simulink subsystem "Sensors"  (R2025a)
settings: Solver=VariableStepAuto  StartTime=0.0  StopTime=10.0  RelTol=1e-3
undefined symbols (not defined in the file): DiscIntNeverNeededParam, gyro_bias0, gyro_bias_rw, gyro_sigma, rng_seed, star_sigma, Ts_base, Ts_gyro, Ts_star
settings Model: Creator=Jackt  LastModifiedBy=Jackt

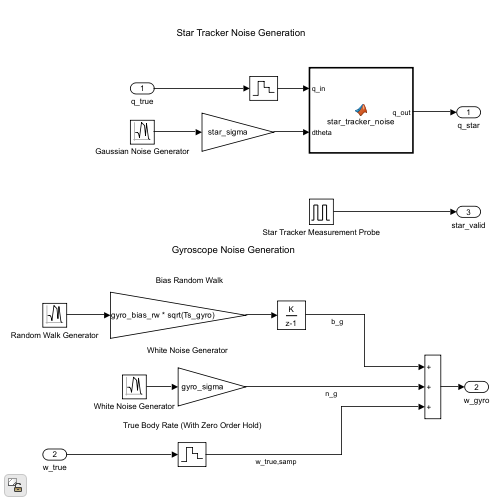
[thumbnail: Simulink's stored preview of the top-level diagram]
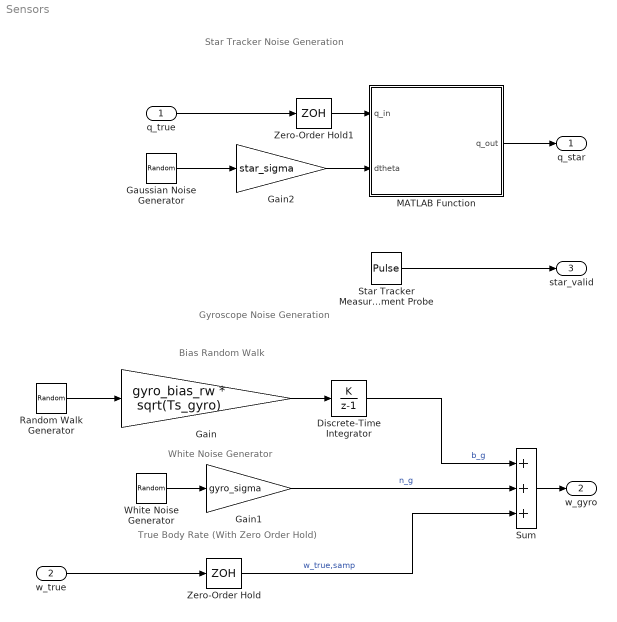
== system Sensors ==
  note: Gyroscope Noise Generation
  note: True Body Rate (With Zero Order Hold)
  note: White Noise Generator
  note: Bias Random Walk
  note: Star Tracker Noise Generation
  q_true : Inport
  w_true : Inport  Port=2
  Discrete-Time Integrator : DiscreteIntegrator  IntegratorMethod=Accumulation: Forward Euler  InitialCondition=gyro_bias0  SampleTime=Ts_gyro  ICPrevOutput=DiscIntNeverNeededParam  ICPrevScaledInput=DiscIntNeverNeededParam
  Gain : Gain  Gain=gyro_bias_rw * sqrt(Ts_gyro)
  Gain1 : Gain  Gain=gyro_sigma
  Gain2 : Gain  Gain=star_sigma
  Gaussian Noise Generator : RandomNumber  Mean=[0; 0; 0]  Variance=[1; 1; 1]  Seed=rng_seed  SampleTime=Ts_star  VectorParams1D=off
  MATLAB Function : MATLAB Function  TreatAsAtomicUnit=on
  Random Walk Generator : RandomNumber  Mean=[0; 0; 0]  Variance=[1; 1; 1]  Seed=rng_seed  SampleTime=Ts_gyro  VectorParams1D=off
  Star Tracker Measurement Probe : DiscretePulseGenerator  PulseType=Time based  Period=Ts_star  PulseWidth=100*Ts_base/Ts_star  VectorParams1D=off
  Sum : Sum  Inputs=+++
  White Noise Generator : RandomNumber  Mean=[0; 0; 0]  Variance=[1; 1; 1]  Seed=rng_seed  SampleTime=Ts_gyro  VectorParams1D=off
  Zero-Order Hold : ZeroOrderHold  SampleTime=Ts_gyro
  Zero-Order Hold1 : ZeroOrderHold  SampleTime=Ts_star
  q_star : Outport
  w_gyro : Outport  Port=2
  star_valid : Outport  Port=3
  wires:
  q_true/1 -> Zero-Order Hold1/1
  w_true/1 -> Zero-Order Hold/1
  Random Walk Generator/1 -> Gain/1
  Gain/1 -> Discrete-Time Integrator/1
  Discrete-Time Integrator/1 -> Sum/1  "b_g"
  White Noise Generator/1 -> Gain1/1
  Gain1/1 -> Sum/2  "n_g"
  Zero-Order Hold/1 -> Sum/3  "w_true,samp"
  Sum/1 -> w_gyro/1
  Gaussian Noise Generator/1 -> Gain2/1
  Zero-Order Hold1/1 -> MATLAB Function/1(q_in)
  Gain2/1 -> MATLAB Function/2(dtheta)
  MATLAB Function/1(q_out) -> q_star/1
  Star Tracker Measurement Probe/1 -> star_valid/1

== matlab function Sensors/MATLAB Function ==
  data: q_in input; q_out output; dtheta input
function q_out = star_tracker_noise(q_in, dtheta)
%STAR_TRACKER_NOISE Apply star-tracker attitude noise to a quaternion.

%Enforce Shapes
q = q_in(:);
d = dtheta(:);

%Input Check
if numel(q) ~= 4 || numel(d) ~= 3 || any(~isfinite(q)) || any(~isfinite(d))
    q_out = [1;0;0;0];
    return;
end

%Normalize Input Quaternions
nq = norm(q);
if nq < 1e-12
    q = [1;0;0;0];
else
    q = q / nq;
end

%Map rotation vector noise to quaternion via exponential map
theta = norm(d);

if theta < 1e-12
    dq = [1;0;0;0];
else
    u = d / theta; %unit axis
    half = 0.5 * theta;
    dq = [cos(half); u * sin(half)];
end

%Measured attitude = true attitude * noise
q_out = quatmultiply_sf(q, dq);

%Normalize output
no = norm(q_out);
if no < 1e-12
    q_out = [1;0;0;0];
else
    q_out = q_out / no;
end

end

function q = quatmultiply_sf(a,b)
%QUATMULTIPLY_SF Scalar-first quaternion multiply: q = a ⊗ b
% a,b,q are [4x1] with scalar first.
w1=a(1); x1=a(2); y1=a(3); z1=a(4);
w2=b(1); x2=b(2); y2=b(3); z2=b(4);

q = [ w1*w2 - x1*x2 - y1*y2 - z1*z2;
      w1*x2 + x1*w2 + y1*z2 - z1*y2;
      w1*y2 - x1*z2 + y1*w2 + z1*x2;
      w1*z2 + x1*y2 - y1*x2 + z1*w2 ];
end
